simulink model "arxeio2teleia4"  (R2021a)
settings: Solver=VariableStepAuto  StartTime=0.0  StopTime=5  RelTol=1e-3
libraries: spsACVoltageSourceLib x3, spsCurrentMeasurementLib x2, spsRMSLib x2, spsAsynchronousMachineSIUnitsLib x1, spsDCVoltageSourceLib x1, simulink x1, spsNeutralLib x1, spsVoltageMeasurementLib x1, spspowerguiLib x1
settings Model: Creator=stama  LastModifiedBy=stama

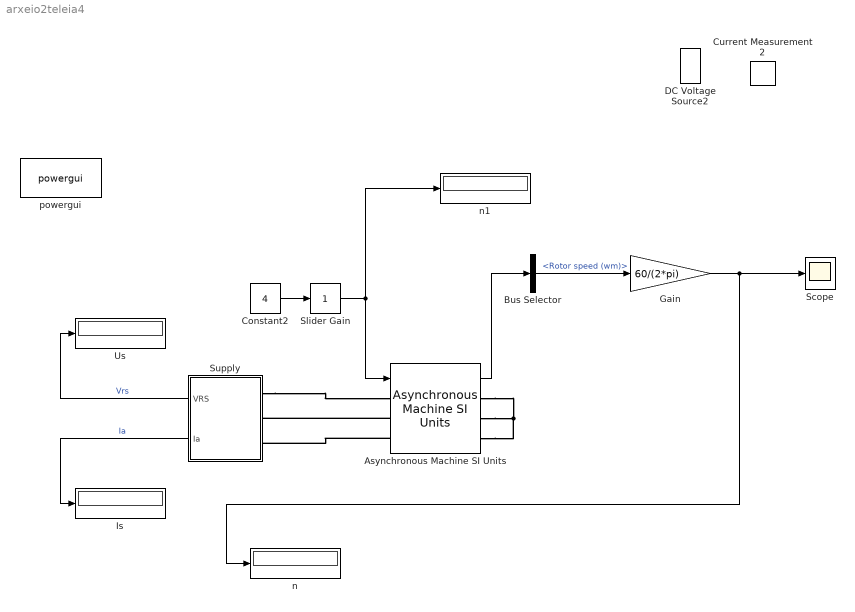
== system arxeio2teleia4 ==
  Asynchronous Machine SI Units : spsAsynchronousMachineSIUnitsLib/Asynchronous Machine SI Units  RotorType=Wound  PresetModel="15:  5.4 HP (4KW)   400 V  50Hz 1430 RPM"  MechanicalLoad=Torque Tm  ShowDetailedParameters=on  ReferenceFrame=Stationary  Units=SI  MeasurementBus=off  NominalParameters=[4000 400 50]  VoltageRatio=1  Stator=[1.405 0.005839]  Rotor=[1.395 0.005839]  Cage1=[0.4155 0.002066]  Cage2=[0.4168 0.0003495]  Lm=0.1722  Mechanical=[0.0131 0.002985 2]  PolePairs=2  InitialConditions=[1 0 0 0 0 0 0 0]  SimulateSaturation=off  Saturation=[14.03593122, 27.81365428, 53.79336849, 72.68890987, 97.98006896, 148.6815601, 215.7428561, 302.9841135, 428.7778367 ; 230, 322, 414, 460, 506, 552, 598, 644, 690]  LoadFlowParameters=1492000  TsPowergui=0  TsBlock=-1  IterativeModel=Trapezoidal non iterative  IterativeDiscreteModel=Trapezoidal non iterative  Pmec=1.492e+006
  Bus Selector : BusSelector  OutputSignals=Mechanical.Rotor speed (wm)
  Constant2 : Constant  Value=4
  Current Measurement2 : spsCurrentMeasurementLib/Current Measurement  PhasorSimulation=off  OutputType=Complex  PSBequivalent=0
  DC Voltage Source2 : spsDCVoltageSourceLib/DC Voltage Source  Amplitude=100  Measurements=None
  Gain : Gain  Gain=60/(2*pi)
  Is : Display
  Scope : Scope
  Slider Gain : simulink/Math Operations/Slider Gain  gain=1  low=0  high=2
  Supply : Subsystem  mask{VLL=100.1}
      mask prompts: VLL "Line Voltage (V)"
      mask DialogControl Label1 Prompt: 3 phase power supply
  Us : Display
  n : Display
  n1 : Display
  powergui : spspowerguiLib/powergui  Priority=1  SimulationMode=Continuous  SampleTime=50e-6  frequency=60  Iterations=50  frequencyindice=50  Pbase=100e6  ErrMax=1e-4  UnitsV=kV  UnitsW=MW  buscounter=0  FunctionMessages=off  echomessages=off  EnableUseOfTLC=off  CurrentSourceSwitches=off  DisableSnubberDevices=off  DisableRonSwitches=off  DisableVfSwitches=off  DisplayEquations=off  AutomaticDiscreteSolvers=off  SolverType=Tustin/Backward Euler (TBE)  Interpol=off  ExternalGateDelay=off  methode=off  Ts=100  x0status=blocks  SPID=on  SwTol=0  HookPort=off  NonlinearTolerance=1e-4  nMaxIteration=100  ContinueOnMaxIteration=off  RestoreLinks=warning  ResistiveCurrentMeasurement=off  Frange=[0:2:500]  Ylog=off  Xlog=on  ShowGrid=off  save=off  variable=ZData  structure=0  ZoomFFT=off  StartTime=0.0  cycles=1  DisplayStyle=1  fundamental=60  FreqAxis=off  MaxFrequency=1000  frequencyindicesteady=1  RmsSteady=1  display=off
  wires:
  Gain/1 -> n/1, Scope/1
  Asynchronous Machine SI Units/1 -> Bus Selector/1
  Supply/1(VRS) -> Us/1  "Vrs"
  Supply/2(Ia) -> Is/1  "Ia"
  Bus Selector/1 -> Gain/1  "<Rotor speed (wm)>"
  Slider Gain/1 -> n1/1, Asynchronous Machine SI Units/1
  Constant2/1 -> Slider Gain/1
  connections:
  Supply/LConn1 -- Asynchronous Machine SI Units/LConn1
  Asynchronous Machine SI Units/LConn2 -- Supply/LConn2
  Asynchronous Machine SI Units/RConn2 -- Asynchronous Machine SI Units/RConn3 -- Asynchronous Machine SI Units/RConn1
  Asynchronous Machine SI Units/LConn3 -- Supply/LConn3

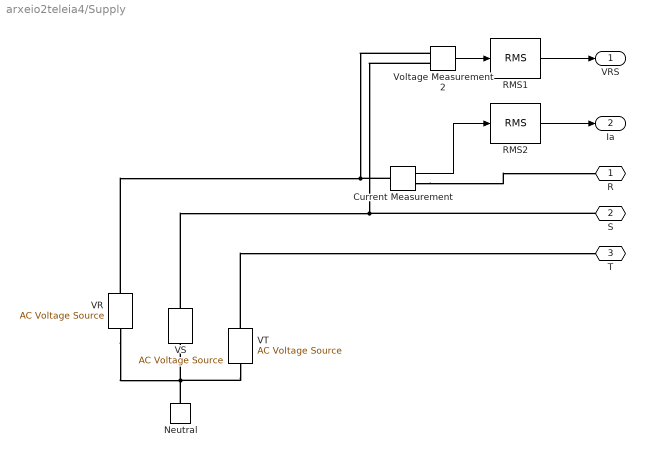
== system arxeio2teleia4/Supply ==
  Current Measurement : spsCurrentMeasurementLib/Current Measurement  PhasorSimulation=off  OutputType=Complex  PSBequivalent=0
  Neutral : spsNeutralLib/Neutral  LConnTagsString=a  NodeNumber=10
      settings: AttributesFormatString=node %<NodeNumber>  SourceProductBaseCode=PS
  RMS1 : spsRMSLib/RMS  TrueRMS=on  Freq=50  RMSInit=0  Ts=0
  RMS2 : spsRMSLib/RMS  TrueRMS=on  Freq=50  RMSInit=0  Ts=0
  VR : spsACVoltageSourceLib/AC Voltage Source  Amplitude=VLL*sqrt(2/3)  Phase=0  Frequency=50  SampleTime=0  Measurements=None  BusType=swing  Pref=10e3  Qref=0  Qmin=-inf  Qmax=+inf
  VS : spsACVoltageSourceLib/AC Voltage Source  Amplitude=VLL*sqrt(2/3)  Phase=-120  Frequency=50  SampleTime=0  Measurements=None  BusType=swing  Pref=10e3  Qref=0  Qmin=-inf  Qmax=+inf
  VT : spsACVoltageSourceLib/AC Voltage Source  Amplitude=VLL*sqrt(2/3)  Phase=120  Frequency=50  SampleTime=0  Measurements=None  BusType=swing  Pref=10e3  Qref=0  Qmin=-inf  Qmax=+inf
  Voltage Measurement2 : spsVoltageMeasurementLib/Voltage Measurement  PhasorSimulation=off  OutputType=Complex  PSBequivalent=0
  R : PMIOPort  Side=Left
  S : PMIOPort  Port=2  Side=Left
  T : PMIOPort  Port=3  Side=Left
  VRS : Outport
  Ia : Outport  Port=2
  wires:
  Voltage Measurement2/1 -> RMS1/1
  RMS1/1 -> VRS/1
  Current Measurement/1 -> RMS2/1
  RMS2/1 -> Ia/1
  connections:
  Current Measurement/RConn1 -- R/RConn1
  Voltage Measurement2/LConn1 -- VR/RConn1 -- Current Measurement/LConn1
  VT/RConn1 -- T/RConn1
  Voltage Measurement2/LConn2 -- VS/RConn1 -- S/RConn1
  VR/LConn1 -- VT/LConn1 -- VS/LConn1 -- Neutral/LConn1
